simulink model "tank_based_pos_pos"  (R2021b)
settings: Solver=ode45  StartTime=0.0  StopTime=30  FixedStep=Ts  MinStep=1e-5  RelTol=1e-5
undefined symbols (not defined in the file): A, A_int, B, Be, beta, Bh_i, Bm, Bs, C, delayT, Dh, Discrete, Dm, Ds, Fc, Ff, Fip, Hd, Hm_init, Hs_init, Jh_i, Ke, Kh, Kh_i, Km, Ks, Mm, Ms, posNoiseVariance, R, Time, tlcAlpha, Ts, xe
libraries: simulink x3, ctrlSharedLib x2, cstblocks x1
settings Model: Creator=simon  LastModifiedBy=miche
settings SolverCC: AlgebraicLoopSolver=LineSearch
settings DebuggingCC: SFMachineParentedDataDiag=warning

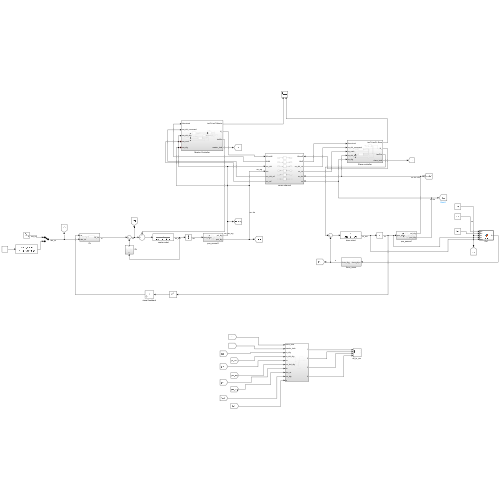
[thumbnail: Simulink's stored preview of the top-level diagram]
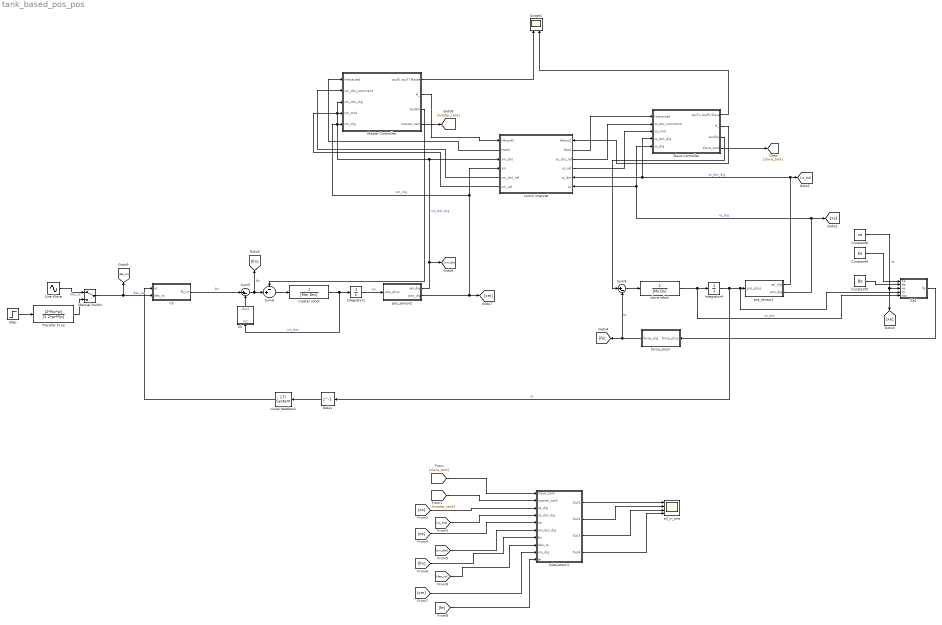
== system tank_based_pos_pos ==
  Ch : Subsystem
  Constant4 : Constant  Value=Ke
  Constant5 : Constant  Value=Be
  Constant6 : Constant  Value=xe
  Delay : Delay  DelayLength=1  SampleTime=Ts
  Integrator1 : Integrator
  Integrator4 : Integrator
  Manual Switch : ManualSwitch
  Master Controller : Subsystem
  Scope1 : Scope  NumInputPorts=2
  Sine Wave : Sin  Amplitude=A_int  Frequency=2*pi*Fc  SampleTime=0
  Slave controller : Subsystem
  Step : Step  SampleTime=0
  Subsystem1 : Subsystem
  Sum5 : Sum  Inputs=|+-
  Sum6 : Sum  Inputs=-+|
  Sum8 : Sum  Inputs=|+-
  Transfer Fcn2 : TransferFcn  Numerator=[2*Fip*pi]  Denominator=[1 2*pi*Fip]
  Ze1 : MATLAB Function  TreatAsAtomicUnit=on
  Zh : Subsystem
  all_in_one : Scope  NumInputPorts=4
  comm channel : Subsystem
      settings: PortSchema="{\"entries\":[{\"content\":{\"sides\":[{\"content\":{\"connectorIds\":[\"In1\",\"Out4\",\"Out5\",\"Out6\",\"In2\",\"In3\"]},\"type\":\"ConnectorPlacement.EquallySpacedRectSide\",\"uuid\":\"1c070cf8-9aa7-4f7b-8e2f-2632c2893f69\"},{\"content\":{\"connectorIds\":[\"In4\",\"Out1\",\"In5\",\"In6\",\"Out2\",\"Out3\"],\"side\":\"RIGHT\"},\"type\":\"ConnectorPlacement.EquallySpacedRectSide\",\"uuid\":\"32173565-3523-4dfc-9820-763c87098354\"},{\"content\":{\"connectorIds\":[],\"side\":\"TOP\"},\"type\":\"ConnectorPlacement.EquallySpacedRectSide\",\"uuid\":\"13187df6-bf6f-436e-a2ee-34150977e6a8\"},{\"content\":{\"connectorIds\":[],\"side\":\"HIDDEN\"},\"type\":\"ConnectorPlacement.EquallySpacedRectSide\",\"uuid\":\"1e5bcdd7-6028-40f7-b524-727817e519ff\"}]},\"type\":\"ConnectorPlacement.EquallySpacedConnector\",\"uuid\":\"c84d0440-83b9-4b92-a10a-1f72bb115b54\"}],\"packageUris\":[\"http://schema.mathworks.com/mf0/Connector/R2020b\"],\"version\":\"1.0\"}"
  force_snsor : Subsystem
  master robot : TransferFcn  Denominator=[Mm Dm]
  pos_sensor1 : Subsystem
  pos_sensor2 : Subsystem
  slave robot : TransferFcn  Denominator=[Ms Ds]
  visual feedback : cstblocks/LTI System  sys=1  IC=[]
  wires:
  Zh/1(Out1) -> Sum5/2
  Integrator1/1 -> pos_sensor2/1(pos_phys)  "xm"
  master robot/1 -> Integrator1/1, Zh/1(In1)  "xm_dot"
  Ch/1(fh_int) -> Sum5/1  "fh*"
  Sum6/1 -> master robot/1
  pos_sensor2/2(pos_dig) -> Master Controller/5(xm_dig), comm channel/6(xm), [xm]  "xm_dig"
  Sum5/1 -> Sum6/2, [fm]  "fm"
  pos_sensor2/1(vel_dig) -> [xm_dot], Master Controller/3(xm_dot_dig), comm channel/5(xm_dot)  "xm_dot_dig"
  slave robot/1 -> Ze1/5(dxs), Integrator4/1  "xs_dot"
  Integrator4/1 -> Ze1/4(xs), pos_sensor1/1(pos_phys), Delay/1  "xs"
  pos_sensor1/2(pos_dig) -> comm channel/3(xs), Slave controller/5(xs_dig), [xs]  "xs_dig"
  pos_sensor1/1(vel_dig) -> Slave controller/4(xs_dot_dig), comm channel/2(xs_dot), [xs_dot]  "xs_dot_dig"
  Sum8/1 -> slave robot/1
  Constant4/1 -> Ze1/1(Ke)
  Constant5/1 -> Ze1/2(Be)
  Constant6/1 -> Ze1/3(xe), [xe]  "xe"
  Ze1/1(fe) -> force_snsor/1(force_phys)
  Manual Switch/1 -> Ch/2(des_xs), [des_xs]  "des_xs"
  visual feedback/1 -> Ch/1(xs)
  Delay/1 -> visual feedback/1
  force_snsor/1(force_dig) -> Sum8/2, [fe]  "fe"
  Transfer Fcn2/1 -> Manual Switch/2
  Step/1 -> Transfer Fcn2/1
  Sine Wave/1 -> Manual Switch/1  "des_xs"
  comm channel/1(HtoM) -> Master Controller/1(Hreceived)
  comm channel/2(xm_dot_ref) -> Master Controller/2(xm_dot_command)
  comm channel/3(xm_ref) -> Master Controller/4(xm_cmd)
  Master Controller/1(tauPL tauTl Master) -> Scope1/1
  Master Controller/2(H_) -> comm channel/4(HfromM)
  Master Controller/3(tauRm) -> Sum6/1
  Master Controller/4(master_tank) -> [master_tank]
  Subsystem1/1(Out1) -> all_in_one/1
  Subsystem1/2(Out2) -> all_in_one/2
  Subsystem1/3(Out3) -> all_in_one/3
  Subsystem1/4(Out4) -> all_in_one/4
  comm channel/4(HtoS) -> Slave controller/1(Hreceived)
  comm channel/5(xs_dot_ref) -> Slave controller/2(xs_dot_command)
  comm channel/6(xs_ref) -> Slave controller/3(xs_cmd)
  Slave controller/1(tauTL tauPL Slave) -> Scope1/2
  Slave controller/2(H_) -> comm channel/1(HfromS)
  Slave controller/3(tauPLs) -> Sum8/1
  Slave controller/4(slave_tank) -> [slave_tank]
  [slave_tank] -> Subsystem1/1(slave_tank)
  [master_tank] -> Subsystem1/2(master_tank)
  [xs] -> Subsystem1/3(xs_dig)
  [xs_dot] -> Subsystem1/4(xs_dot_dig)
  [xe] -> Subsystem1/5(xe)
  [xm_dot] -> Subsystem1/6(xm_dot_dig)
  [fm] -> Subsystem1/7(fm)
  [xm] -> Subsystem1/9(xm_dig)
  [fe] -> Subsystem1/10(fe)
  [des_xs] -> Subsystem1/8(des_xs)

== system tank_based_pos_pos/Ch ==
  xs : Inport
  des_xs : Inport  Port=2
  Sum : Sum  Inputs=|-+
  Transfer Fcn : TransferFcn  Numerator=[Dh Kh]  Denominator=[1 0]
  fh_int : Outport
  wires:
  xs/1 -> Sum/1
  des_xs/1 -> Sum/2
  Sum/1 -> Transfer Fcn/1
  Transfer Fcn/1 -> fh_int/1

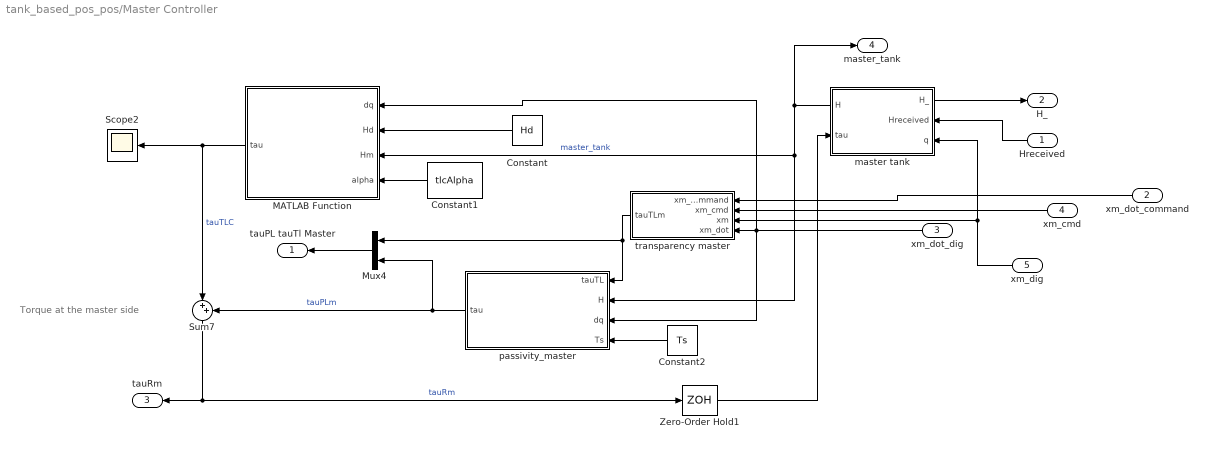
== system tank_based_pos_pos/Master Controller ==
  note: Torque at the master side
  Hreceived : Inport
  xm_dot_command : Inport  Port=2
  xm_dot_dig : Inport  Port=3
  xm_cmd : Inport  Port=4
  xm_dig : Inport  Port=5
  Constant : Constant  Value=Hd
  Constant1 : Constant  Value=tlcAlpha
  Constant2 : Constant  Value=Ts
  MATLAB Function : MATLAB Function  TreatAsAtomicUnit=on
  Mux4 : Mux  Inputs=2
  Scope2 : Scope
  Sum7 : Sum  Inputs=|++
  Zero-Order Hold1 : ZeroOrderHold  SampleTime=Ts
  master tank : Subsystem
      settings: PortSchema="{\"entries\":[{\"content\":{\"sides\":[{\"content\":{\"connectorIds\":[\"Out2\",\"In1\",\"In2\"]},\"type\":\"ConnectorPlacement.EquallySpacedRectSide\",\"uuid\":\"482b0a11-f044-49fa-a74d-4dac8b5b787b\"},{\"content\":{\"connectorIds\":[\"Out1\",\"In3\"],\"side\":\"RIGHT\"},\"type\":\"ConnectorPlacement.EquallySpacedRectSide\",\"uuid\":\"b0c369ed-ae40-43d8-b393-bca9f7720d62\"},{\"content\":{\"connectorIds\":[],\"side\":\"TOP\"},\"type\":\"ConnectorPlacement.EquallySpacedRectSide\",\"uuid\":\"ff021616-d6aa-4c0a-874b-a9ebe947c92c\"},{\"content\":{\"connectorIds\":[],\"side\":\"BOTTOM\"},\"type\":\"ConnectorPlacement.EquallySpacedRectSide\",\"uuid\":\"4e18ee96-bca7-41b6-9abb-5b593b41c296\"},{\"content\":{\"connectorIds\":[],\"side\":\"HIDDEN\"},\"type\":\"ConnectorPlacement.EquallySpacedRectSide\",\"uuid\":\"be815b34-35c7-4c6f-8c8b-4a812b3d12e9\"}]},\"type\":\"ConnectorPlacement.EquallySpacedConnector\",\"uuid\":\"78552b8a-5f1c-4815-a807-de98f58b7f2e\"}],\"packageUris\":[\"http://schema.mathworks.com/mf0/Connector/R2020b\"],\"version\":\"1.0\"}"
  passivity_master : MATLAB Function  TreatAsAtomicUnit=on
  transparency master : Subsystem
  tauPL tauTl Master : Outport
  H_ : Outport  Port=2
  tauRm : Outport  Port=3
  master_tank : Outport  Port=4
  wires:
  master tank/1(H) -> MATLAB Function/3(Hm), passivity_master/2(H), master_tank/1  "master_tank"
  Constant2/1 -> passivity_master/4(Ts)
  MATLAB Function/1(tau) -> Sum7/1, Scope2/1  "tauTLC"
  Sum7/1 -> Zero-Order Hold1/1, tauRm/1  "tauRm"
  Constant/1 -> MATLAB Function/2(Hd)
  Mux4/1 -> tauPL tauTl Master/1
  transparency master/1(tauTLm) -> passivity_master/1(tauTL), Mux4/1
  xm_cmd/1 -> transparency master/2(xm_cmd)
  passivity_master/1(tau) -> Mux4/2, Sum7/2  "tauPLm"
  Zero-Order Hold1/1 -> master tank/3(tau)
  Constant1/1 -> MATLAB Function/4(alpha)
  Hreceived/1 -> master tank/1(Hreceived)
  master tank/2(H_) -> H_/1
  xm_dig/1 -> master tank/2(q), transparency master/3(xm)
  xm_dot_dig/1 -> passivity_master/3(dq), MATLAB Function/1(dq), transparency master/4(xm_dot)
  xm_dot_command/1 -> transparency master/1(xm_dot_command)

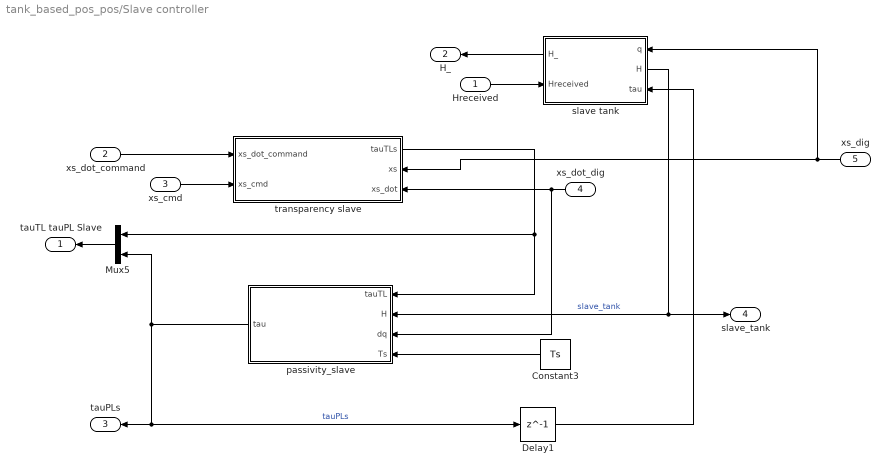
== system tank_based_pos_pos/Slave controller ==
  Hreceived : Inport
  xs_dot_command : Inport  Port=2
  xs_cmd : Inport  Port=3
  xs_dot_dig : Inport  Port=4
  xs_dig : Inport  Port=5
  Constant3 : Constant  Value=Ts
  Delay1 : Delay  DelayLength=1  SampleTime=Ts
  Mux5 : Mux  Inputs=2
  passivity_slave : MATLAB Function  TreatAsAtomicUnit=on
  slave tank : Subsystem
      settings: PortSchema="{\"entries\":[{\"content\":{\"sides\":[{\"content\":{\"connectorIds\":[\"In1\",\"Out2\",\"In2\"]},\"type\":\"ConnectorPlacement.EquallySpacedRectSide\",\"uuid\":\"482b0a11-f044-49fa-a74d-4dac8b5b787b\"},{\"content\":{\"connectorIds\":[\"Out1\",\"In3\"],\"side\":\"RIGHT\"},\"type\":\"ConnectorPlacement.EquallySpacedRectSide\",\"uuid\":\"b0c369ed-ae40-43d8-b393-bca9f7720d62\"},{\"content\":{\"connectorIds\":[],\"side\":\"TOP\"},\"type\":\"ConnectorPlacement.EquallySpacedRectSide\",\"uuid\":\"ff021616-d6aa-4c0a-874b-a9ebe947c92c\"},{\"content\":{\"connectorIds\":[],\"side\":\"BOTTOM\"},\"type\":\"ConnectorPlacement.EquallySpacedRectSide\",\"uuid\":\"4e18ee96-bca7-41b6-9abb-5b593b41c296\"},{\"content\":{\"connectorIds\":[],\"side\":\"HIDDEN\"},\"type\":\"ConnectorPlacement.EquallySpacedRectSide\",\"uuid\":\"be815b34-35c7-4c6f-8c8b-4a812b3d12e9\"}]},\"type\":\"ConnectorPlacement.EquallySpacedConnector\",\"uuid\":\"78552b8a-5f1c-4815-a807-de98f58b7f2e\"}],\"packageUris\":[\"http://schema.mathworks.com/mf0/Connector/R2020b\"],\"version\":\"1.0\"}"
  transparency slave : Subsystem
      settings: PortSchema="{\"entries\":[{\"content\":{\"sides\":[{\"content\":{\"connectorIds\":[\"In1\",\"In2\"]},\"type\":\"ConnectorPlacement.EquallySpacedRectSide\",\"uuid\":\"c8f256d1-8287-4bc6-9264-40c0684f6acd\"},{\"content\":{\"connectorIds\":[\"Out1\",\"In3\",\"In4\"],\"side\":\"RIGHT\"},\"type\":\"ConnectorPlacement.EquallySpacedRectSide\",\"uuid\":\"cb9f571e-93fc-426e-a4f2-aa96ae3bd6b3\"},{\"content\":{\"connectorIds\":[],\"side\":\"TOP\"},\"type\":\"ConnectorPlacement.EquallySpacedRectSide\",\"uuid\":\"b9b91304-f20e-4a66-aa64-b99c686ee85a\"},{\"content\":{\"connectorIds\":[],\"side\":\"HIDDEN\"},\"type\":\"ConnectorPlacement.EquallySpacedRectSide\",\"uuid\":\"c3abcf5a-e3b9-4b9a-a4b1-68c5725be1f4\"}]},\"type\":\"ConnectorPlacement.EquallySpacedConnector\",\"uuid\":\"83907002-acbd-4948-aeba-a43201e13c19\"}],\"packageUris\":[\"http://schema.mathworks.com/mf0/Connector/R2020b\"],\"version\":\"1.0\"}"
  tauTL tauPL Slave : Outport
  H_ : Outport  Port=2
  tauPLs : Outport  Port=3
  slave_tank : Outport  Port=4
  wires:
  xs_dig/1 -> slave tank/1(q), transparency slave/3(xs)
  transparency slave/1(tauTLs) -> Mux5/1, passivity_slave/1(tauTL)
  xs_dot_dig/1 -> passivity_slave/3(dq), transparency slave/4(xs_dot)
  Hreceived/1 -> slave tank/3(Hreceived)
  passivity_slave/1(tau) -> Mux5/2, Delay1/1, tauPLs/1  "tauPLs"
  Constant3/1 -> passivity_slave/4(Ts)
  Delay1/1 -> slave tank/2(tau)
  slave tank/2(H) -> slave_tank/1, passivity_slave/2(H)  "slave_tank"
  xs_dot_command/1 -> transparency slave/1(xs_dot_command)
  xs_cmd/1 -> transparency slave/2(xs_cmd)
  Mux5/1 -> tauTL tauPL Slave/1
  slave tank/1(H_) -> H_/1

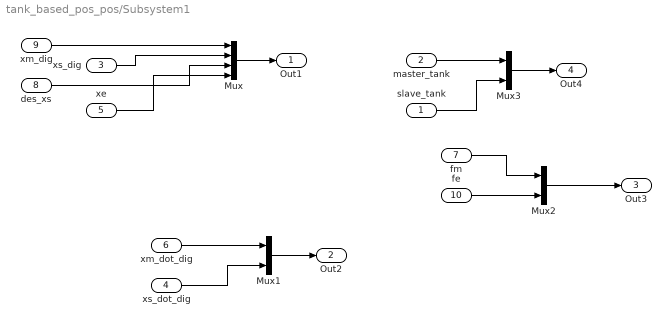
== system tank_based_pos_pos/Subsystem1 ==
  slave_tank : Inport
  master_tank : Inport  Port=2
  xs_dig : Inport  Port=3
  xs_dot_dig : Inport  Port=4
  xe : Inport  Port=5
  xm_dot_dig : Inport  Port=6
  fm : Inport  Port=7
  des_xs : Inport  Port=8
  xm_dig : Inport  Port=9
  fe : Inport  Port=10
  Mux : Mux
  Mux1 : Mux  Inputs=2
  Mux2 : Mux  Inputs=2
  Mux3 : Mux  Inputs=2
  Out1 : Outport
  Out2 : Outport  Port=2
  Out3 : Outport  Port=3
  Out4 : Outport  Port=4
  wires:
  fe/1 -> Mux2/2
  Mux/1 -> Out1/1
  xm_dig/1 -> Mux/1
  xe/1 -> Mux/4
  xm_dot_dig/1 -> Mux1/1
  slave_tank/1 -> Mux3/2
  fm/1 -> Mux2/1
  master_tank/1 -> Mux3/1
  Mux1/1 -> Out2/1
  Mux2/1 -> Out3/1
  xs_dot_dig/1 -> Mux1/2
  Mux3/1 -> Out4/1
  des_xs/1 -> Mux/3
  xs_dig/1 -> Mux/2

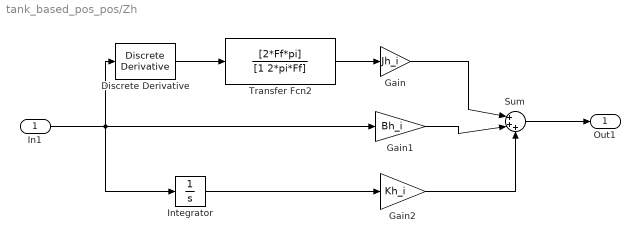
== system tank_based_pos_pos/Zh ==
  In1 : Inport
  Discrete Derivative : simulink/Discrete/Discrete Derivative  gainval=1.0  ICPrevScaledInput=0.0  OutMin=[]  OutMax=[]  OutDataType=fixdt(1, 16)  OutScaling=2^-10  DoSatur=off
  Gain : Gain  Gain=Jh_i
  Gain1 : Gain  Gain=Bh_i
  Gain2 : Gain  Gain=Kh_i
  Integrator : Integrator
  Sum : Sum  Inputs=|+++
  Transfer Fcn2 : TransferFcn  Numerator=[2*Ff*pi]  Denominator=[1 2*pi*Ff]
  Out1 : Outport
  wires:
  Integrator/1 -> Gain2/1
  In1/1 -> Gain1/1, Integrator/1, Discrete Derivative/1
  Gain/1 -> Sum/1
  Gain1/1 -> Sum/2
  Gain2/1 -> Sum/3
  Sum/1 -> Out1/1
  Discrete Derivative/1 -> Transfer Fcn2/1
  Transfer Fcn2/1 -> Gain/1

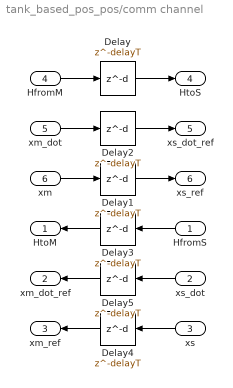
== system tank_based_pos_pos/comm channel ==
  HfromS : Inport
  xs_dot : Inport  Port=2
  xs : Inport  Port=3
  HfromM : Inport  Port=4
  xm_dot : Inport  Port=5
  xm : Inport  Port=6
  Delay{,1..5} (6 alike) : Delay  DelayLength=delayT  SampleTime=Ts
  HtoM : Outport
  xm_dot_ref : Outport  Port=2
  xm_ref : Outport  Port=3
  HtoS : Outport  Port=4
  xs_dot_ref : Outport  Port=5
  xs_ref : Outport  Port=6
  wires:
  HfromS/1 -> Delay3/1
  xm_dot/1 -> Delay2/1
  xm/1 -> Delay1/1
  Delay1/1 -> xs_ref/1
  Delay2/1 -> xs_dot_ref/1
  HfromM/1 -> Delay/1
  Delay/1 -> HtoS/1
  Delay3/1 -> HtoM/1
  Delay4/1 -> xm_ref/1
  Delay5/1 -> xm_dot_ref/1
  xs_dot/1 -> Delay5/1
  xs/1 -> Delay4/1

== system tank_based_pos_pos/force_snsor ==
  force_phys : Inport
  Sum5 : Sum  Inputs=|++
  Transfer Fcn : TransferFcn  Commented=on  Numerator=[2*Fip*pi]  Denominator=[1 2*pi*Fip]
  Zero-Order Hold1 : ZeroOrderHold  SampleTime=Ts
  sensor noise : RandomNumber  Commented=on  Variance=0.0000001  SampleTime=Ts
  force_dig : Outport
  wires:
  force_phys/1 -> Zero-Order Hold1/1
  sensor noise/1 -> Sum5/2
  Zero-Order Hold1/1 -> Sum5/1
  Sum5/1 -> force_dig/1  "force_dig"

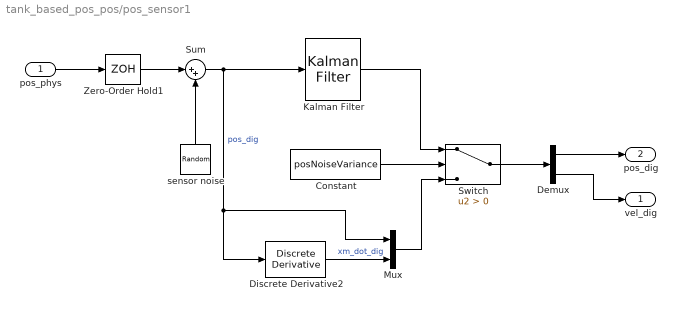
== system tank_based_pos_pos/pos_sensor1 ==
  pos_phys : Inport
  Constant : Constant  Value=posNoiseVariance
  Demux : Demux  Outputs=2
  Discrete Derivative2 : simulink/Discrete/Discrete Derivative  gainval=1.0  ICPrevScaledInput=0.0  OutMin=[]  OutMax=[]  OutDataType=fixdt(1, 16)  OutScaling=2^-10  DoSatur=off
  Kalman Filter : ctrlSharedLib/Kalman Filter  TimeDomain=Discrete-Time  UseCurrentEstimator=on  ModelSource=Individual A, B, C, D matrices  ModelSourceVariable=ss(0.95,1,1,0,1)  A=A  B=B  C=C  D=0  NumberOfStates=2  NumberOfInputs=1  NumberOfOutputs=1  InitialEstimateSource=Dialog  X0=0  P0=10  UseK=off  UseGH=off  NumberOfProcessNoiseInputs=1  G=1  TimeInvariantG=on  H=0  TimeInvariantH=on  Q=Q_m  TimeInvariantQ=on  R=R  TimeInvariantR=on  N=0  TimeInvariantN=on  AddInputPort=off  AddEnablePort=off  OutputEstimatedY=off  OutputP=off  Ts=Ts
  Mux : Mux  Inputs=2
  Sum : Sum  Inputs=|++
  Switch : Switch  Criteria=u2 > Threshold
  Zero-Order Hold1 : ZeroOrderHold  SampleTime=Ts
  sensor noise : RandomNumber  Variance=posNoiseVariance  SampleTime=Ts
  vel_dig : Outport
  pos_dig : Outport  Port=2
  wires:
  pos_phys/1 -> Zero-Order Hold1/1
  Zero-Order Hold1/1 -> Sum/1
  sensor noise/1 -> Sum/2
  Kalman Filter/1 -> Switch/1
  Sum/1 -> Mux/1, Discrete Derivative2/1, Kalman Filter/1  "pos_dig"
  Constant/1 -> Switch/2
  Mux/1 -> Switch/3
  Discrete Derivative2/1 -> Mux/2  "xm_dot_dig"
  Switch/1 -> Demux/1
  Demux/1 -> pos_dig/1
  Demux/2 -> vel_dig/1

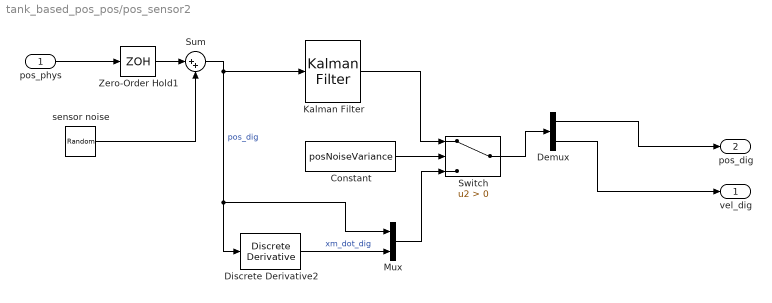
== system tank_based_pos_pos/pos_sensor2 ==
  pos_phys : Inport
  Constant : Constant  Value=posNoiseVariance
  Demux : Demux  Outputs=2
  Discrete Derivative2 : simulink/Discrete/Discrete Derivative  gainval=1.0  ICPrevScaledInput=0.0  OutMin=[]  OutMax=[]  OutDataType=fixdt(1, 16)  OutScaling=2^-10  DoSatur=off
  Kalman Filter : ctrlSharedLib/Kalman Filter  TimeDomain=Discrete-Time  UseCurrentEstimator=on  ModelSource=Individual A, B, C, D matrices  ModelSourceVariable=ss(0.95,1,1,0,1)  A=A  B=B  C=C  D=0  NumberOfStates=2  NumberOfInputs=1  NumberOfOutputs=1  InitialEstimateSource=Dialog  X0=0  P0=10  UseK=off  UseGH=off  NumberOfProcessNoiseInputs=1  G=1  TimeInvariantG=on  H=0  TimeInvariantH=on  Q=Q_m  TimeInvariantQ=on  R=R  TimeInvariantR=on  N=0  TimeInvariantN=on  AddInputPort=off  AddEnablePort=off  OutputEstimatedY=off  OutputP=off  Ts=Ts
  Mux : Mux  Inputs=2
  Sum : Sum  Inputs=|++
  Switch : Switch  Criteria=u2 > Threshold
  Zero-Order Hold1 : ZeroOrderHold  SampleTime=Ts
  sensor noise : RandomNumber  Variance=posNoiseVariance  SampleTime=Ts
  vel_dig : Outport
  pos_dig : Outport  Port=2
  wires:
  pos_phys/1 -> Zero-Order Hold1/1
  Zero-Order Hold1/1 -> Sum/1
  sensor noise/1 -> Sum/2
  Kalman Filter/1 -> Switch/1
  Sum/1 -> Mux/1, Discrete Derivative2/1, Kalman Filter/1  "pos_dig"
  Constant/1 -> Switch/2
  Mux/1 -> Switch/3
  Discrete Derivative2/1 -> Mux/2  "xm_dot_dig"
  Switch/1 -> Demux/1
  Demux/1 -> pos_dig/1
  Demux/2 -> vel_dig/1

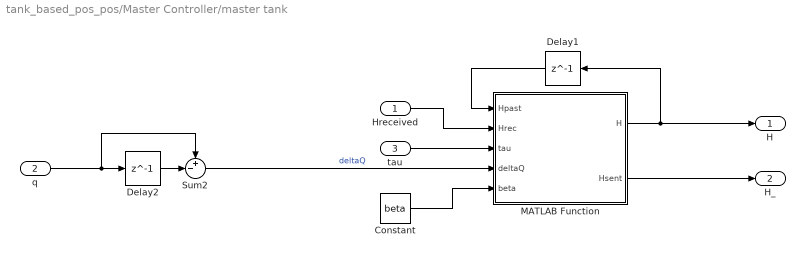
== system tank_based_pos_pos/Master Controller/master tank ==
  Hreceived : Inport
  q : Inport  Port=2
  tau : Inport  Port=3
  Constant : Constant  Value=beta
  Delay1 : Delay  DelayLength=1  InitialCondition=Hm_init  SampleTime=Ts
  Delay2 : Delay  DelayLength=1  SampleTime=Ts
  MATLAB Function : MATLAB Function  TreatAsAtomicUnit=on
  Sum2 : Sum  Inputs=+-|
  H : Outport
  H_ : Outport  Port=2
  wires:
  Delay2/1 -> Sum2/2
  q/1 -> Delay2/1, Sum2/1
  MATLAB Function/2(Hsent) -> H_/1
  Constant/1 -> MATLAB Function/5(beta)
  Sum2/1 -> MATLAB Function/4(deltaQ)  "deltaQ"
  Hreceived/1 -> MATLAB Function/2(Hrec)
  tau/1 -> MATLAB Function/3(tau)
  MATLAB Function/1(H) -> Delay1/1, H/1
  Delay1/1 -> MATLAB Function/1(Hpast)

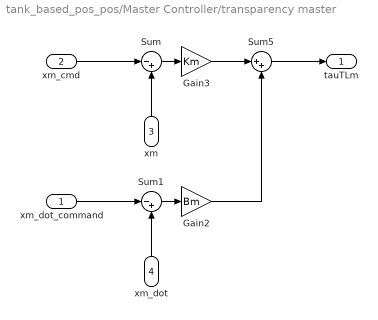
== system tank_based_pos_pos/Master Controller/transparency master ==
  xm_dot_command : Inport
  xm_cmd : Inport  Port=2
  xm : Inport  Port=3
  xm_dot : Inport  Port=4
  Gain2 : Gain  Gain=Bm
  Gain3 : Gain  Gain=Km
  Sum : Sum  Inputs=|-+
  Sum1 : Sum  Inputs=|-+
  Sum5 : Sum  Inputs=|++
  tauTLm : Outport
  wires:
  Sum5/1 -> tauTLm/1
  Sum/1 -> Gain3/1
  Sum1/1 -> Gain2/1
  Gain3/1 -> Sum5/1
  xm_dot_command/1 -> Sum1/1
  Gain2/1 -> Sum5/2
  xm/1 -> Sum/2
  xm_dot/1 -> Sum1/2
  xm_cmd/1 -> Sum/1

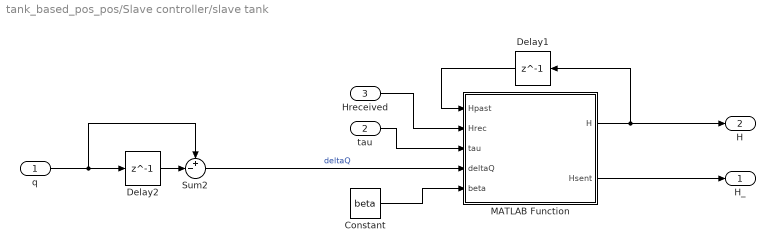
== system tank_based_pos_pos/Slave controller/slave tank ==
  q : Inport
  tau : Inport  Port=2
  Hreceived : Inport  Port=3
  Constant : Constant  Value=beta
  Delay1 : Delay  DelayLength=1  InitialCondition=Hs_init  SampleTime=Ts
  Delay2 : Delay  DelayLength=1  SampleTime=Ts
  MATLAB Function : MATLAB Function  TreatAsAtomicUnit=on
  Sum2 : Sum  Inputs=+-|
  H_ : Outport
  H : Outport  Port=2
  wires:
  Delay2/1 -> Sum2/2
  q/1 -> Delay2/1, Sum2/1
  MATLAB Function/2(Hsent) -> H_/1
  Constant/1 -> MATLAB Function/5(beta)
  Sum2/1 -> MATLAB Function/4(deltaQ)  "deltaQ"
  Hreceived/1 -> MATLAB Function/2(Hrec)
  tau/1 -> MATLAB Function/3(tau)
  MATLAB Function/1(H) -> Delay1/1, H/1
  Delay1/1 -> MATLAB Function/1(Hpast)

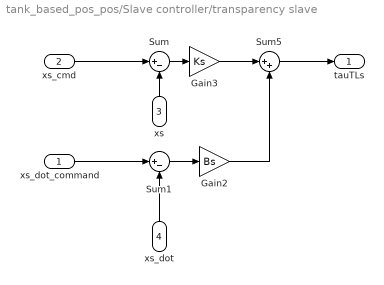
== system tank_based_pos_pos/Slave controller/transparency slave ==
  xs_dot_command : Inport
  xs_cmd : Inport  Port=2
  xs : Inport  Port=3
  xs_dot : Inport  Port=4
  Gain2 : Gain  Gain=Bs
  Gain3 : Gain  Gain=Ks
  Sum : Sum  Inputs=|+-
  Sum1 : Sum  Inputs=|+-
  Sum5 : Sum  Inputs=|++
  tauTLs : Outport
  wires:
  Sum5/1 -> tauTLs/1
  xs_cmd/1 -> Sum/1
  xs_dot_command/1 -> Sum1/1
  Gain2/1 -> Sum5/2
  Gain3/1 -> Sum5/1
  Sum/1 -> Gain3/1
  Sum1/1 -> Gain2/1
  xs/1 -> Sum/2
  xs_dot/1 -> Sum1/2

== matlab function tank_based_pos_pos/Master Controller/MATLAB Function ==
  data: dq input; tau output; Hd input; Hm input; alpha input
function tau = tauTLC(dq, Hd, Hm, alpha)
%tank level controller
%Energy Tanks slide 16
if Hd <= Hm
    d = 0;
else
    d = alpha*(Hd-Hm);
end
tau = -d*dq;

== matlab function tank_based_pos_pos/Master Controller/master tank/MATLAB Function ==
  data: Hpast input; H output; Hrec input; tau input; deltaQ input; beta input; Hsent output
function [H,Hsent] = tank(Hpast, Hrec, tau, deltaQ, beta)

Hused = tau*deltaQ;
H = Hpast+Hrec-Hused;    
Hsent = H*beta;

%H(k+1)
H = H-Hsent;

== matlab function tank_based_pos_pos/Slave controller/slave tank/MATLAB Function ==
  data: Hpast input; H output; Hrec input; tau input; deltaQ input; beta input; Hsent output
function [H,Hsent] = tank(Hpast, Hrec, tau, deltaQ, beta)
Hused = tau*deltaQ;
H = Hpast+Hrec-Hused;    
Hsent = H*beta;
H = H-Hsent;

== matlab function tank_based_pos_pos/Slave controller/passivity_slave ==
  data: tauTL input; H input; tau output; dq input; Ts input
function tau = tauPL(tauTL, H, dq,Ts)

%saturation and control torque 
%slide 19 tau max 1 2

if H<= 0
    tauMax1 = 0;
else
    tauMax1 = tauTL;
end
tauMax2 = H/(dq*Ts);
%limited torque computed by the passivity layer based on τauTL
tau = sign(tauTL)*min([abs(tauMax1),abs(tauMax2)]);

== matlab function tank_based_pos_pos/Master Controller/passivity_master ==
  data: tauTL input; H input; tau output; dq input; Ts input
function tau = tauPL(tauTL, H, dq,Ts)
%saturation and control torque 
%slide 19 tau max 1 2
if H<= 0
    tauMax1 = 0;
else
    tauMax1 = tauTL;
end
tauMax2 = H/(dq*Ts);

%limited torque computed by the passivity layer based on τauTL
tau = sign(tauTL)*min([abs(tauMax1),abs(tauMax2)]);

== matlab function tank_based_pos_pos/Ze1 ==
  data: Ke input; fe output; Be input; xe input; xs input; dxs input
function fe = env(Ke, Be, xe, xs, dxs)
    if xs > xe
        fe = Ke*(xs-xe)+Be*max(dxs, 0);
    else
        fe = 0;
    end
